simulink model "Three_torques_inputs"  (R2015a)
settings: Solver=ode45  SolverMode=SingleTasking  StartTime=0.0  StopTime=20  MaxStep=0.01  RelTol=1e-3
values from neighbouring files (symbols this model uses):
  A = eval(As)    [Three_torque_input.m]    (also in matlab.mat = [0 0 0 1 0 0 0 0 0 0 1 0 ... (36 elements, 6x6)])
  B = eval(Bs)    [Three_torque_input.m]    (also in matlab.mat = [7142857.14286 0 0 0 0 0 0 7142857.14286 0 0 0 0 ... (18 ele)
  Cs = [1 0 0 0 0 0; 0 1 0 0 0 0; 0 0 1 0 0 0;  0 0 0 1 0 0;0 0 0 0 1 0]    [Three_torque_input.m]    (also in matlab.mat = [1 0 0 0 0 0 1 0 0 0 0 0 ... (30 elements, 5x6)])
  Kd = [9.34671886994e-07 6.22367483075e-14 2.77863544329e-15 6.22275735362e-14 9.34671962103e-07 -1.84446499623e-18 4.28409489953e-15 -2.86027102975e-18 3.07145457868e-06 3.12004941218e-06 1.38412246569e-13 7.35162501932e-15 ... (15 elements, 3x5)]    [matlab.mat]
  Kr_d = -inv(Cc*inv(Aa-Bb*Kd-eye(5))*Bb)    [Three_torque_input.m]    (also in matlab.mat = [4.28409489953e-15  3.12004941218e-06  1.33824860896e-13; -2)
  ts = 1/250    (= 0.004)    [Three_torque_input.m]    (also in matlab.mat)
libraries: dspsigops x2
settings Model: Creator=Jaby  LastModifiedBy=Jaby
settings OptimizationCC: BlockReduction=off  BooleanDataType=off
settings DebuggingCC: SaveWithParameterizedLinksMsg=none  UnderspecifiedInitializationDetection=Classic  MergeDetectMultiDrivingBlocksExec=none  SignalResolutionControl=TryResolveAllWithWarning
settings HardwareCC: TargetUnknown=on

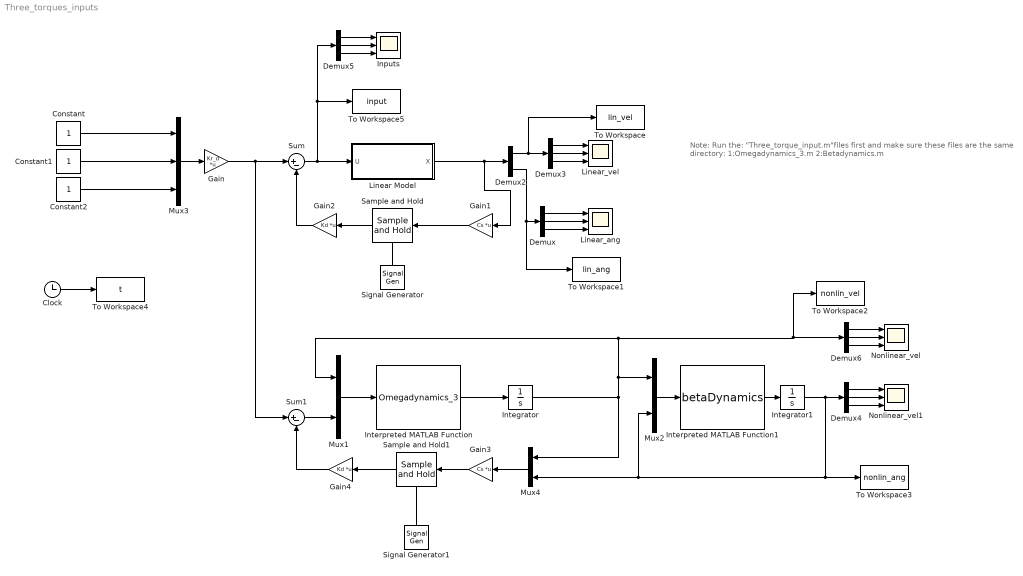
== system Three_torques_inputs ==
  note: Note:
      | Run the: "Three_torque_input.m"files first
      | and make sure these files are the same directory:
      | 1:Omegadynamics_3.m
      | 2:Betadynamics.m
  Clock : Clock
  Constant : Constant
  Constant1 : Constant
  Constant2 : Constant
  Demux{,3..6} (5 alike) : Demux  Outputs=3
  Demux2 : Demux  Outputs=2
  Gain : Gain  Gain=Kr_d  Multiplication=Matrix(K*u)
  Gain1 : Gain  Gain=Cs  Multiplication=Matrix(K*u)
  Gain2 : Gain  Gain=Kd  Multiplication=Matrix(K*u)
  Gain3 : Gain  Gain=Cs  Multiplication=Matrix(K*u)
  Gain4 : Gain  Gain=Kd  Multiplication=Matrix(K*u)
  Inputs : Scope  NumInputPorts=3
      settings: TimeRange=20  YMin=0~0~-1  YMax=2e+07~7000~1  SaveName=ScopeData4
  Integrator : Integrator  InitialCondition=[0 0 0]'
  Integrator1 : Integrator  InitialCondition=[0 0 0]'
  Interpreted MATLAB Function : MATLABFcn  MATLABFcn=Omegadynamics_3  Output1D=off
  Interpreted MATLAB Function1 : MATLABFcn  MATLABFcn=betaDynamics  Output1D=off
  "Linear Model " : Subsystem
  Linear_ang : Scope  NumInputPorts=3
      settings: TimeRange=20  YMin=0.00274~-3.07e-14~8.3e-31  YMax=0.00278~-3.025e-14~8.430000000000001e-31
  Linear_vel : Scope  NumInputPorts=3
      settings: TimeRange=20  YMin=0~0~-1  YMax=2e+07~7000~1  SaveName=ScopeData2
  Mux1 : Mux  Inputs=2
  Mux2 : Mux  Inputs=2
  Mux3 : Mux  Inputs=3
  Mux4 : Mux  Inputs=2
  Nonlinear_vel : Scope  NumInputPorts=3
      settings: TimeRange=20  YMin=0~0~-1  YMax=2e+07~7000~1  SaveName=ScopeData5
  Nonlinear_vel1 : Scope  NumInputPorts=3
      settings: TimeRange=20  YMin=0~0~-1  YMax=2e+07~7000~1  SaveName=ScopeData3
  Sample and Hold : dspsigops/Sample and Hold  trig=Rising edge  initCond=0  latchinput=off
  Sample and Hold1 : dspsigops/Sample and Hold  trig=Rising edge  initCond=0  latchinput=off
  Signal Generator : SignalGenerator  WaveForm=square  Frequency=1/ts  VectorParams1D=off
  Signal Generator1 : SignalGenerator  WaveForm=square  Frequency=1/ts  VectorParams1D=off
  Sum : Sum  Inputs=|+-
  Sum1 : Sum  Inputs=|+-
  To Workspace : ToWorkspace  VariableName=lin_vel  SampleTime=-1
  To Workspace1 : ToWorkspace  VariableName=lin_ang  SampleTime=-1
  To Workspace2 : ToWorkspace  VariableName=nonlin_vel  SampleTime=-1
  To Workspace3 : ToWorkspace  VariableName=nonlin_ang  SampleTime=-1
  To Workspace4 : ToWorkspace  VariableName=t  SampleTime=-1
  To Workspace5 : ToWorkspace  VariableName=input  SampleTime=-1
  wires:
  "Linear Model "/1(X) -> Gain1/1, Demux2/1
  Demux/1 -> Linear_ang/1
  Demux/2 -> Linear_ang/2
  Demux/3 -> Linear_ang/3
  Mux1/1 -> Interpreted MATLAB Function/1
  Interpreted MATLAB Function/1 -> Integrator/1
  Interpreted MATLAB Function1/1 -> Integrator1/1
  Mux2/1 -> Interpreted MATLAB Function1/1
  Demux2/2 -> To Workspace1/1, Demux/1
  Demux3/1 -> Linear_vel/1
  Demux3/2 -> Linear_vel/2
  Demux3/3 -> Linear_vel/3
  Demux2/1 -> To Workspace/1, Demux3/1
  Mux3/1 -> Gain/1
  Clock/1 -> To Workspace4/1
  Gain/1 -> Sum1/1, Sum/1
  Demux5/2 -> Inputs/2
  Demux5/3 -> Inputs/3
  Demux5/1 -> Inputs/1
  Sum/1 -> Demux5/1, To Workspace5/1, "Linear Model "/1(U)
  Gain2/1 -> Sum/2
  Constant/1 -> Mux3/1
  Constant1/1 -> Mux3/2
  Constant2/1 -> Mux3/3
  Mux4/1 -> Gain3/1
  Sum1/1 -> Mux1/2
  Gain4/1 -> Sum1/2
  Demux6/1 -> Nonlinear_vel/1
  Demux6/2 -> Nonlinear_vel/2
  Demux6/3 -> Nonlinear_vel/3
  Integrator/1 -> Mux4/1, To Workspace2/1, Demux6/1, Mux1/1, Mux2/1
  Demux4/1 -> Nonlinear_vel1/1
  Demux4/2 -> Nonlinear_vel1/2
  Demux4/3 -> Nonlinear_vel1/3
  Integrator1/1 -> Demux4/1, Mux2/2, Mux4/2, To Workspace3/1
  Gain1/1 -> Sample and Hold/1
  Sample and Hold/1 -> Gain2/1
  Signal Generator/1 -> Sample and Hold/Trigger
  Signal Generator1/1 -> Sample and Hold1/Trigger
  Gain3/1 -> Sample and Hold1/1
  Sample and Hold1/1 -> Gain4/1

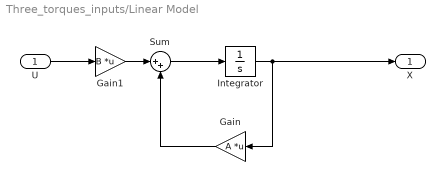
== system Three_torques_inputs/Linear Model  ==
  U : Inport
  Gain : Gain  Gain=A  Multiplication=Matrix(K*u)
  Gain1 : Gain  Gain=B  Multiplication=Matrix(K*u)
  Integrator : Integrator
  Sum : Sum  Inputs=|++
  X : Outport
  wires:
  Integrator/1 -> X/1, Gain/1
  U/1 -> Gain1/1
  Gain1/1 -> Sum/1
  Sum/1 -> Integrator/1
  Gain/1 -> Sum/2
